simulink model "correlation"  (R2024b)
settings: Solver=FixedStepDiscrete  StartTime=0.0  StopTime=30  RelTol=1e-3
InitFcn:
  | % Define a random matrix size between 3 and 10
  | n =4;
  | 
  | fprintf('Size of matrix A: n = %d\n', n);
libraries: simulink x1
settings Model: DataTypeOverride=Off  Creator=valen  LastModifiedBy=valen
settings SolverCC: AlgebraicLoopSolver=TrustRegion
settings DataIOCC: LimitDataPoints=on  SaveOutput=off  SaveTime=off
settings OptimizationCC: BlockReduction=off  ConditionallyExecuteInputs=off  DefaultParameterBehavior=Inlined  LifeSpan=inf
settings DebuggingCC: AlgebraicLoopMsg=error  SingleTaskRateTransMsg=error  UnconnectedInputMsg=warning  UnconnectedOutputMsg=warning  UnconnectedLineMsg=warning  AllowSymbolicDim=off  StrictBusMsg=ErrorOnBusTreatedAsVector  SFUnexpectedBacktrackingDiag=warning  SFNoUnconditionalDefaultTransitionDiag=warning  SFExecutionAtInitializationDiag=none  ArithmeticOperatorsInVariantConditions=warning
settings HardwareCC: ProdBitPerPointer=32  ProdBitPerSizeT=32  ProdBitPerPtrDiffT=32  ProdLargestAtomicFloat=None  ProdIntDivRoundTo=Undefined  ProdEndianess=Unspecified  ProdWordSize=32  ProdHWDeviceType=ASIC/FPGA->ASIC/FPGA  ProdEqTarget=off
settings ModelReferenceCC: EnableRefExpFcnMdlSchedulingChecks=on
settings SFSimCC: SimUseLocalCustomCode=off  CustomCodeUndefinedFunction=UseInterfaceOnly
settings RTWCC: RTWUseLocalCustomCode=off  GPUComputeCapability=3.5
settings CodeAppCC: StateflowObjectComments=on
settings GRTTargetCC: TargetLangStandard=C89/C90 (ANSI)
settings ConfigComp: CovScope=ReferencedModels  CovMetricSettings=dw  CovSaveCumulativeToWorkspaceVar=on  CovSaveSingleToWorkspaceVar=on  CovExternalEMLEnable=off  CovSFcnEnable=off

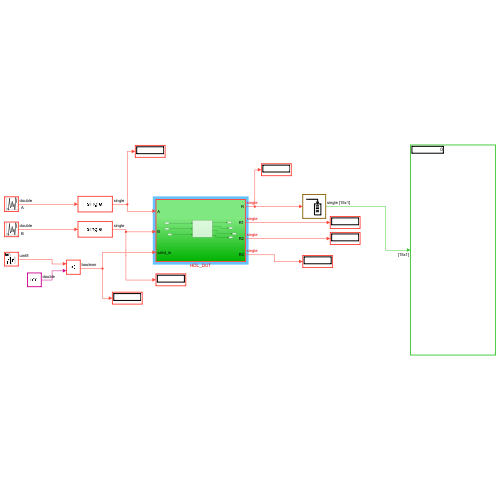
[thumbnail: Simulink's stored preview of the top-level diagram]
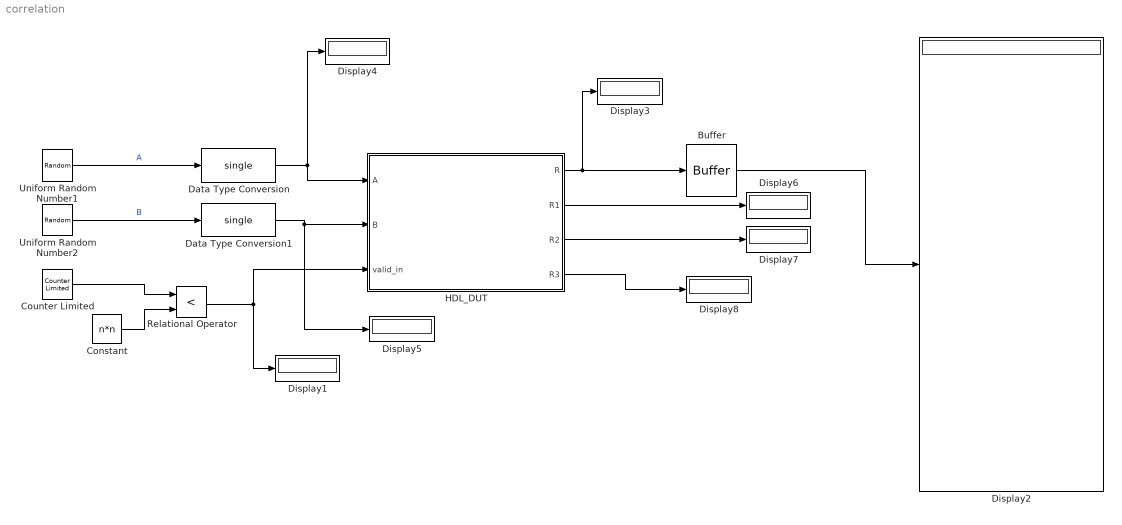
== system correlation ==
  Buffer : Buffer  N=15  OutputFrames=off
  Constant : Constant  Value=n*n
  Counter Limited : simulink/Sources/Counter Limited  uplimit=n*(n+1)  tsamp=-1
  Data Type Conversion : DataTypeConversion  OutDataTypeStr=single  SaturateOnIntegerOverflow=off  RndMeth=Floor
  Data Type Conversion1 : DataTypeConversion  OutDataTypeStr=single  SaturateOnIntegerOverflow=off  RndMeth=Floor
  Display{1..8} (8 alike) : Display
  HDL_DUT : Subsystem
  Relational Operator : RelationalOperator  Operator=<  OutDataTypeStr=boolean  RndMeth=Simplest  InputSameDT=off
  Uniform Random Number1 : UniformRandomNumber  Minimum=0  Maximum=5  Seed=n  SampleTime=10/(n*n+1)
  Uniform Random Number2 : UniformRandomNumber  Minimum=0  Maximum=5  Seed=n  SampleTime=10/(n*n+1)
  wires:
  HDL_DUT/1(R) -> Buffer/1, Display3/1
  Uniform Random Number1/1 -> Data Type Conversion/1  "A"
  Buffer/1 -> Display2/1
  Data Type Conversion/1 -> Display4/1, HDL_DUT/1(A)
  Counter Limited/1 -> Relational Operator/1
  Constant/1 -> Relational Operator/2
  Relational Operator/1 -> HDL_DUT/3(valid_in), Display1/1
  Uniform Random Number2/1 -> Data Type Conversion1/1  "B"
  Data Type Conversion1/1 -> Display5/1, HDL_DUT/2(B)
  HDL_DUT/2(R1) -> Display6/1
  HDL_DUT/3(R2) -> Display7/1
  HDL_DUT/4(R3) -> Display8/1

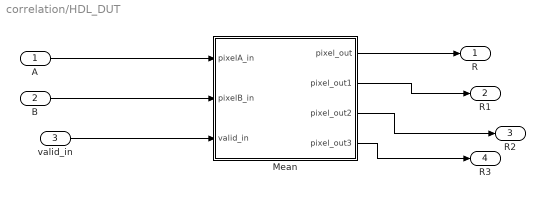
== system correlation/HDL_DUT ==
  A : Inport
  B : Inport  Port=2
  valid_in : Inport  Port=3
  Mean : MATLAB Function  TreatAsAtomicUnit=on
  R : Outport  VectorParamsAs1DForOutWhenUnconnected=off
  R1 : Outport  Port=2  VectorParamsAs1DForOutWhenUnconnected=off
  R2 : Outport  Port=3  VectorParamsAs1DForOutWhenUnconnected=off
  R3 : Outport  Port=4  VectorParamsAs1DForOutWhenUnconnected=off
  wires:
  Mean/1(pixel_out) -> R/1
  valid_in/1 -> Mean/3(valid_in)
  A/1 -> Mean/1(pixelA_in)
  B/1 -> Mean/2(pixelB_in)
  Mean/2(pixel_out1) -> R1/1
  Mean/3(pixel_out2) -> R2/1
  Mean/4(pixel_out3) -> R3/1

== matlab function correlation/HDL_DUT/Mean ==
  data: pixelA_in input; pixelB_in input; pixel_out output; valid_in input; pixel_out1 output; pixel_out2 output; pixel_out3 output
function [pixel_out, pixel_out1, pixel_out2, pixel_out3] = hardware_softmax(pixelA_in, pixelB_in, valid_in)
    % Constantes fixes (Taille 2x2 = 4 pixels)
    TOTAL_PIXELS = int32(16);
    INV_TOTAL    = single(0.25); % Remplacer la division par une multiplication (Plus léger en hardware)
    
    % Registres persistants (Mémoires et États FSM)
    persistent bufferA bufferB;
    persistent meanA meanB;
    persistent sum_diffA2 sum_diffB2 sum_cross;
    persistent count state;
    
    % Initialisation unique des variables persistantes
    if isempty(state)
        bufferA     = zeros(1, 16, 'single');
        bufferB     = zeros(1, 16, 'single');
        meanA       = single(0);
        meanB       = single(0);
        sum_diffA2  = single(0);
        sum_diffB2  = single(0);
        sum_cross   = single(0);
        count       = int32(1);
        state       = int32(0); 
    end
    
    % Initialisation des sorties par défaut (Évite les verrous d'incompatibilité/latches)
    pixel_out  = single(0);
    pixel_out1 = single(0);
    pixel_out2 = single(0);
    pixel_out3 = single(0);
    
    % Machine à états (FSM)
    switch state
        case 0 % --- ÉTAPE 1 : ACQUISITION DU FLUX ---
            if valid_in
                bufferA(count) = pixelA_in;
                bufferB(count) = pixelB_in;
                
                if count == TOTAL_PIXELS
                    count = int32(1);
                    state = int32(1); % Matrice complète, passage au calcul
                else
                    count = count + 1;
                end
            end
            
        case 1 % --- ÉTAPE 2 : CALCUL DES MOYENNES (Parallèle) ---
            % Utilisation de sum() sur tout le vecteur d'un coup (Arbre d'addition parallèle)
            meanA = sum(bufferA) * INV_TOTAL; 
            meanB = sum(bufferB) * INV_TOTAL;
            state = int32(2);
            
        case 2 % --- ÉTAPE 3 : ARBRE DE CALCUL DES DIFFÉRENCES ET PRODUITS ---
            % CORRECTION HARDWARE : Pour éviter les feedback-loops au fil de l'eau,
            % on vectorise l'opération sur la petite window de 4 éléments.
            % HDL Coder transformera cela en pure logique combinatoire parallèle sans boucles.
            diffA = bufferA - meanA;
            diffB = bufferB - meanB;
            
            % Calculs des variances et covariance
            sum_diffA2 = sum(diffA .* diffA);
            sum_diffB2 = sum(diffB .* diffB);
            sum_cross  = sum(diffA .* diffB);
            
            state = int32(3);
            
        case 3 % --- ÉTAPE 4 : OPÉRATION LOURDE (Pipeline Vivado) ---
            % HDL Coder insérera automatiquement les registres nécessaires pour la racine 
            % carrée et la division grâce au pipeline.
            denom = sqrt(sum_diffA2 * sum_diffB2);
            
            if denom > 0.0
                pixel_out = sum_cross / denom;
            else
                pixel_out = single(0);
            end
            
            % Assignation des sorties finales
            pixel_out1 = sum_cross
            pixel_out2 = sum_diffA2
            pixel_out3 = sum_diffB2
            
            % Reset complet des accumulateurs pour la prochaine matrice
            meanA      = single(0);
            meanB      = single(0);
            sum_cross  = single(0);
            sum_diffA2 = single(0);
            sum_diffB2 = single(0);
            count      = int32(1);
            state      = int32(0); % Retour à l'écoute des entrées
    end
end
